simulink model "Integration"  (R2024b)
settings: Solver=VariableStepAuto  StartTime=0.0  StopTime=4  RelTol=1e-3
undefined symbols (not defined in the file): Ion, Lithium, Ts_Control
libraries: spsSeriesRLCBranchLib x37, ee_lib x30, nesl_utility x30, spsCurrentVoltageSimscapeInterfaceLib x18, slpidlib x9, spsThreePhaseVIMeasurementLib x7, spsParallelRLCBranchLib x7, spsThreePhaseSeriesRLCBranchLib x7, spsGroundLib x7, spsDiodeLib x6, spsIGBTDiodeLib x6, spsPWMGeneratorDCDCLib x6
(part 4 of 4)

== matlab function Integration/Subsystem13/MPPT/MATLAB Function1 ==
  data: ipv input; D output; vpv input
function D = mppt_inccond_pi(ipv, vpv)
    % Combined INC MPPT + PI Voltage Controller for Boost Converter
    % Inputs:
    %   ipv - PV current (A)
    %   vpv - PV voltage (V)
    % Output:
    %   D   - Duty cycle (0 < D < 1)

    % Persistent variables to store previous states
    persistent I_prev V_prev Vpv_ref_prev integral_err D_prev

    % Initialize persistent variables
    if isempty(I_prev)
        I_prev = ipv;
        V_prev = vpv;
        Vpv_ref_prev = 360;     % Initial guess near Vmpp
        integral_err = 0;
        D_prev = 0.4;           % Mid-range initial duty
    end

    % === MPPT: Incremental Conductance ===
    delta_Vpv = 1.5;           % Step size for Vpv_ref adjustment
    tol = 1e-4;                % MPP detection tolerance
    v_min = 5;                 % Minimum voltage threshold

    if isnan(ipv) || isnan(vpv) || vpv < v_min
        D = D_prev;
        return;
    end

    delta_I = ipv - I_prev;
    delta_V = vpv - V_prev;

    if abs(delta_V) < 1e-4
        if delta_I > 1e-3
            Vpv_ref = Vpv_ref_prev + delta_Vpv;
        elseif delta_I < -1e-3
            Vpv_ref = Vpv_ref_prev - delta_Vpv;
        else
            Vpv_ref = Vpv_ref_prev;
        end
    else
        inst_cond = ipv / vpv;
        inc_cond = delta_I / delta_V;

        if abs(inc_cond + inst_cond) < tol
            Vpv_ref = Vpv_ref_prev;
        elseif inc_cond > -inst_cond
            Vpv_ref = Vpv_ref_prev + delta_Vpv;
        else
            Vpv_ref = Vpv_ref_prev - delta_Vpv;
        end
    end

    % Clamp Vpv_ref to safe range
    Vpv_ref = min(426.5, max(150, Vpv_ref));

    % === PI Controller to Track Vpv_ref ===
    Kp = 0.09;                 % Proportional gain
    Ki = 15;                   % Integral gain
    Ts = 1e-3;                 % Sampling time (adjust as needed)

    error = (Vpv_ref - vpv) / Vpv_ref;  % Normalized error

    integral_err = integral_err + error * Ts;

    % PI output (raw duty)
    D = Kp * error + Ki * integral_err;

    % Clamp duty cycle
    D_min = 0.43;
    D_max = 0.51;
    D = max(D_min, min(D_max, D));

    % Anti-windup: stop integrating if saturated
    if D == D_min || D == D_max
        integral_err = integral_err - error * Ts;
    end

    % Update states
    I_prev = ipv;
    V_prev = vpv;
    Vpv_ref_prev = Vpv_ref;
    D_prev = D;
end

== matlab function Integration/Subsystem13/MPPT/MATLAB Function2 ==
  data: ipv input; D output; vpv input
function D = inccond_mppt(ipv, vpv)
    % Incremental Conductance MPPT algorithm for PV system (optimized for boost converter)
    % Inputs: ipv - PV current (A), vpv - PV voltage (V)
    % Output: D - Duty cycle (0.2 to 0.392)

    persistent I_prev V_prev D_prev;
    if isempty(I_prev)
        I_prev = 0;
        V_prev = 0; % Initial PV voltage (based on Vmp = 364.5 V)
        D_prev = 0; % Initial duty cycle
    end

    delta_D = 0.008; % Step size for duty cycle adjustment
    D_min = 0.391;     % Minimum duty cycle
    D_max = 0.48;     % Maximum duty cycle
    tol = 1e-3;      % Tolerance for MPP detection
    v_min = 1e-3;    % Minimum voltage threshold

    % Check for invalid inputs
    if isnan(ipv) || isnan(vpv) || ipv < 0 || vpv < v_min
        D = D_prev;
        return;
    end

    % Calculate incremental changes
    delta_I = ipv - I_prev;
    delta_V = vpv - V_prev;

    % Handle small delta_V
    if abs(delta_V) < 1e-4
        if delta_I > 1e-4
            D = D_prev - delta_D; % Increase voltage (decrease D for boost)
        elseif delta_I < -1e-4
            D = D_prev + delta_D; % Decrease voltage (increase D for boost)
        else
            D = D_prev; % No change
        end
    else
        % Calculate instantaneous and incremental conductance
        inst_cond = ipv / vpv; % I/V
        inc_cond = delta_I / delta_V; % dI/dV

        % Compare incremental and instantaneous conductance
        if abs(inc_cond + inst_cond) < tol
            D = D_prev; % At MPP
        elseif inc_cond > -inst_cond
            D = D_prev - delta_D; % Left of MPP, increase voltage (decrease D for boost)
        else
            D = D_prev + delta_D; % Right of MPP, decrease voltage (increase D for boost)
        end
    end

    % Limit duty cycle
    D = min(D_max, max(D_min, D));

    % Update previous values
    I_prev = ipv;
    V_prev = vpv;
    D_prev = D;
end

== matlab function Integration/Subsystem15/MPPT/MATLAB Function1 ==
  data: ipv input; D output; vpv input
function D = mppt_inccond_pi(ipv, vpv)
    % Combined INC MPPT + PI Voltage Controller for Boost Converter
    % Inputs:
    %   ipv - PV current (A)
    %   vpv - PV voltage (V)
    % Output:
    %   D   - Duty cycle (0 < D < 1)

    % Persistent variables to store previous states
    persistent I_prev V_prev Vpv_ref_prev integral_err D_prev

    % Initialize persistent variables
    if isempty(I_prev)
        I_prev = ipv;
        V_prev = vpv;
        Vpv_ref_prev = 360;     % Initial guess near Vmpp
        integral_err = 0;
        D_prev = 0.4;           % Mid-range initial duty
    end

    % === MPPT: Incremental Conductance ===
    delta_Vpv = 1.5;           % Step size for Vpv_ref adjustment
    tol = 1e-4;                % MPP detection tolerance
    v_min = 5;                 % Minimum voltage threshold

    if isnan(ipv) || isnan(vpv) || vpv < v_min
        D = D_prev;
        return;
    end

    delta_I = ipv - I_prev;
    delta_V = vpv - V_prev;

    if abs(delta_V) < 1e-4
        if delta_I > 1e-3
            Vpv_ref = Vpv_ref_prev + delta_Vpv;
        elseif delta_I < -1e-3
            Vpv_ref = Vpv_ref_prev - delta_Vpv;
        else
            Vpv_ref = Vpv_ref_prev;
        end
    else
        inst_cond = ipv / vpv;
        inc_cond = delta_I / delta_V;

        if abs(inc_cond + inst_cond) < tol
            Vpv_ref = Vpv_ref_prev;
        elseif inc_cond > -inst_cond
            Vpv_ref = Vpv_ref_prev + delta_Vpv;
        else
            Vpv_ref = Vpv_ref_prev - delta_Vpv;
        end
    end

    % Clamp Vpv_ref to safe range
    Vpv_ref = min(426.5, max(150, Vpv_ref));

    % === PI Controller to Track Vpv_ref ===
    Kp = 0.09;                 % Proportional gain
    Ki = 15;                   % Integral gain
    Ts = 1e-3;                 % Sampling time (adjust as needed)

    error = (Vpv_ref - vpv) / Vpv_ref;  % Normalized error

    integral_err = integral_err + error * Ts;

    % PI output (raw duty)
    D = Kp * error + Ki * integral_err;

    % Clamp duty cycle
    D_min = 0.57;
    D_max = 0.64;
    D = max(D_min, min(D_max, D));

    % Anti-windup: stop integrating if saturated
    if D == D_min || D == D_max
        integral_err = integral_err - error * Ts;
    end

    % Update states
    I_prev = ipv;
    V_prev = vpv;
    Vpv_ref_prev = Vpv_ref;
    D_prev = D;
end

== matlab function Integration/Subsystem15/MPPT/MATLAB Function2 ==
  data: ipv input; D output; vpv input
function D = inccond_mppt(ipv, vpv)
    % Incremental Conductance MPPT algorithm for PV system (optimized for boost converter)
    % Inputs: ipv - PV current (A), vpv - PV voltage (V)
    % Output: D - Duty cycle (0.2 to 0.392)

    persistent I_prev V_prev D_prev;
    if isempty(I_prev)
        I_prev = 0;
        V_prev = 0; % Initial PV voltage (based on Vmp = 364.5 V)
        D_prev = 0; % Initial duty cycle
    end

    delta_D = 0.008; % Step size for duty cycle adjustment
    D_min = 0.391;     % Minimum duty cycle
    D_max = 0.48;     % Maximum duty cycle
    tol = 1e-3;      % Tolerance for MPP detection
    v_min = 1e-3;    % Minimum voltage threshold

    % Check for invalid inputs
    if isnan(ipv) || isnan(vpv) || ipv < 0 || vpv < v_min
        D = D_prev;
        return;
    end

    % Calculate incremental changes
    delta_I = ipv - I_prev;
    delta_V = vpv - V_prev;

    % Handle small delta_V
    if abs(delta_V) < 1e-4
        if delta_I > 1e-4
            D = D_prev - delta_D; % Increase voltage (decrease D for boost)
        elseif delta_I < -1e-4
            D = D_prev + delta_D; % Decrease voltage (increase D for boost)
        else
            D = D_prev; % No change
        end
    else
        % Calculate instantaneous and incremental conductance
        inst_cond = ipv / vpv; % I/V
        inc_cond = delta_I / delta_V; % dI/dV

        % Compare incremental and instantaneous conductance
        if abs(inc_cond + inst_cond) < tol
            D = D_prev; % At MPP
        elseif inc_cond > -inst_cond
            D = D_prev - delta_D; % Left of MPP, increase voltage (decrease D for boost)
        else
            D = D_prev + delta_D; % Right of MPP, decrease voltage (increase D for boost)
        end
    end

    % Limit duty cycle
    D = min(D_max, max(D_min, D));

    % Update previous values
    I_prev = ipv;
    V_prev = vpv;
    D_prev = D;
end

== matlab function Integration/Subsystem18/MPPT/MATLAB Function1 ==
  data: ipv input; D output; vpv input
function D = mppt_inccond_pi(ipv, vpv)
    % Combined INC MPPT + PI Voltage Controller for Boost Converter
    % Inputs:
    %   ipv - PV current (A)
    %   vpv - PV voltage (V)
    % Output:
    %   D   - Duty cycle (0 < D < 1)

    % Persistent variables to store previous states
    persistent I_prev V_prev Vpv_ref_prev integral_err D_prev

    % Initialize persistent variables
    if isempty(I_prev)
        I_prev = ipv;
        V_prev = vpv;
        Vpv_ref_prev = 360;     % Initial guess near Vmpp
        integral_err = 0;
        D_prev = 0.4;           % Mid-range initial duty
    end

    % === MPPT: Incremental Conductance ===
    delta_Vpv = 1.5;           % Step size for Vpv_ref adjustment
    tol = 1e-4;                % MPP detection tolerance
    v_min = 5;                 % Minimum voltage threshold

    if isnan(ipv) || isnan(vpv) || vpv < v_min
        D = D_prev;
        return;
    end

    delta_I = ipv - I_prev;
    delta_V = vpv - V_prev;

    if abs(delta_V) < 1e-4
        if delta_I > 1e-3
            Vpv_ref = Vpv_ref_prev + delta_Vpv;
        elseif delta_I < -1e-3
            Vpv_ref = Vpv_ref_prev - delta_Vpv;
        else
            Vpv_ref = Vpv_ref_prev;
        end
    else
        inst_cond = ipv / vpv;
        inc_cond = delta_I / delta_V;

        if abs(inc_cond + inst_cond) < tol
            Vpv_ref = Vpv_ref_prev;
        elseif inc_cond > -inst_cond
            Vpv_ref = Vpv_ref_prev + delta_Vpv;
        else
            Vpv_ref = Vpv_ref_prev - delta_Vpv;
        end
    end

    % Clamp Vpv_ref to safe range
    Vpv_ref = min(426.5, max(150, Vpv_ref));

    % === PI Controller to Track Vpv_ref ===
    Kp = 0.09;                 % Proportional gain
    Ki = 15;                   % Integral gain
    Ts = 1e-3;                 % Sampling time (adjust as needed)

    error = (Vpv_ref - vpv) / Vpv_ref;  % Normalized error

    integral_err = integral_err + error * Ts;

    % PI output (raw duty)
    D = Kp * error + Ki * integral_err;

    % Clamp duty cycle
    D_min = 0.72;
    D_max = 0.76;
    D = max(D_min, min(D_max, D));

    % Anti-windup: stop integrating if saturated
    if D == D_min || D == D_max
        integral_err = integral_err - error * Ts;
    end

    % Update states
    I_prev = ipv;
    V_prev = vpv;
    Vpv_ref_prev = Vpv_ref;
    D_prev = D;
end

== matlab function Integration/Subsystem/MPPT/MATLAB Function1 ==
  data: ipv input; D output; vpv input
function D = mppt_inccond_pi(ipv, vpv)
    % Combined INC MPPT + PI Voltage Controller for Boost Converter
    % Inputs:
    %   ipv - PV current (A)
    %   vpv - PV voltage (V)
    % Output:
    %   D   - Duty cycle (0 < D < 1)

    % Persistent variables to store previous states
    persistent I_prev V_prev Vpv_ref_prev integral_err D_prev

    % Initialize persistent variables
    if isempty(I_prev)
        I_prev = ipv;
        V_prev = vpv;
        Vpv_ref_prev = 360;     % Initial guess near Vmpp
        integral_err = 0;
        D_prev = 0.4;           % Mid-range initial duty
    end

    % === MPPT: Incremental Conductance ===
    delta_Vpv = 1.5;           % Step size for Vpv_ref adjustment
    tol = 1e-4;                % MPP detection tolerance
    v_min = 5;                 % Minimum voltage threshold

    if isnan(ipv) || isnan(vpv) || vpv < v_min
        D = D_prev;
        return;
    end

    delta_I = ipv - I_prev;
    delta_V = vpv - V_prev;

    if abs(delta_V) < 1e-4
        if delta_I > 1e-3
            Vpv_ref = Vpv_ref_prev + delta_Vpv;
        elseif delta_I < -1e-3
            Vpv_ref = Vpv_ref_prev - delta_Vpv;
        else
            Vpv_ref = Vpv_ref_prev;
        end
    else
        inst_cond = ipv / vpv;
        inc_cond = delta_I / delta_V;

        if abs(inc_cond + inst_cond) < tol
            Vpv_ref = Vpv_ref_prev;
        elseif inc_cond > -inst_cond
            Vpv_ref = Vpv_ref_prev + delta_Vpv;
        else
            Vpv_ref = Vpv_ref_prev - delta_Vpv;
        end
    end

    % Clamp Vpv_ref to safe range
    Vpv_ref = min(426.5, max(150, Vpv_ref));

    % === PI Controller to Track Vpv_ref ===
    Kp = 0.09;                 % Proportional gain
    Ki = 15;                   % Integral gain
    Ts = 1e-3;                 % Sampling time (adjust as needed)

    error = (Vpv_ref - vpv) / Vpv_ref;  % Normalized error

    integral_err = integral_err + error * Ts;

    % PI output (raw duty)
    D = Kp * error + Ki * integral_err;

    % Clamp duty cycle
    D_min = 0.2;
    D_max = 0.9;
    D = max(D_min, min(D_max, D));

    % Anti-windup: stop integrating if saturated
    if D == D_min || D == D_max
        integral_err = integral_err - error * Ts;
    end

    % Update states
    I_prev = ipv;
    V_prev = vpv;
    Vpv_ref_prev = Vpv_ref;
    D_prev = D;
end

== matlab function Integration/Subsystem18/MPPT/MATLAB Function2 ==
  data: ipv input; D output; vpv input
function D = inccond_mppt(ipv, vpv)
    % Incremental Conductance MPPT algorithm for PV system (optimized for boost converter)
    % Inputs: ipv - PV current (A), vpv - PV voltage (V)
    % Output: D - Duty cycle (0.2 to 0.392)

    persistent I_prev V_prev D_prev;
    if isempty(I_prev)
        I_prev = 0;
        V_prev = 0; % Initial PV voltage (based on Vmp = 364.5 V)
        D_prev = 0; % Initial duty cycle
    end

    delta_D = 0.008; % Step size for duty cycle adjustment
    D_min = 0.391;     % Minimum duty cycle
    D_max = 0.48;     % Maximum duty cycle
    tol = 1e-3;      % Tolerance for MPP detection
    v_min = 1e-3;    % Minimum voltage threshold

    % Check for invalid inputs
    if isnan(ipv) || isnan(vpv) || ipv < 0 || vpv < v_min
        D = D_prev;
        return;
    end

    % Calculate incremental changes
    delta_I = ipv - I_prev;
    delta_V = vpv - V_prev;

    % Handle small delta_V
    if abs(delta_V) < 1e-4
        if delta_I > 1e-4
            D = D_prev - delta_D; % Increase voltage (decrease D for boost)
        elseif delta_I < -1e-4
            D = D_prev + delta_D; % Decrease voltage (increase D for boost)
        else
            D = D_prev; % No change
        end
    else
        % Calculate instantaneous and incremental conductance
        inst_cond = ipv / vpv; % I/V
        inc_cond = delta_I / delta_V; % dI/dV

        % Compare incremental and instantaneous conductance
        if abs(inc_cond + inst_cond) < tol
            D = D_prev; % At MPP
        elseif inc_cond > -inst_cond
            D = D_prev - delta_D; % Left of MPP, increase voltage (decrease D for boost)
        else
            D = D_prev + delta_D; % Right of MPP, decrease voltage (increase D for boost)
        end
    end

    % Limit duty cycle
    D = min(D_max, max(D_min, D));

    % Update previous values
    I_prev = ipv;
    V_prev = vpv;
    D_prev = D;
end
